simulink model "ModelLoadCell"  (R2020b)
settings: Solver=FixedStepAuto  StartTime=0.0  StopTime=10.0  FixedStep=0.010  RelTol=1e-3
settings Model: Creator=kaebi  LastModifiedBy=kaebi

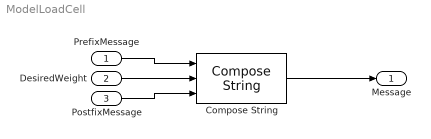
== system ModelLoadCell ==
  PrefixMessage : Inport  OutDataTypeStr=string
  DesiredWeight : Inport  Port=2
  PostfixMessage : Inport  Port=3  OutDataTypeStr=string
  Compose String : ComposeString  Format="\"%s %.3f %s\""
  Message : Outport  OutDataTypeStr=string
  wires:
  DesiredWeight/1 -> Compose String/2
  Compose String/1 -> Message/1
  PostfixMessage/1 -> Compose String/3
  PrefixMessage/1 -> Compose String/1
